simulink model "Thesis_VehicleModel_MPC_ECMS"  (R2018b)
settings: Solver=FixedStepAuto  StartTime=0.0  StopTime=10  FixedStep=0.01  RelTol=1e-5
PostLoadFcn:
  | , if any(exist('dsrtsu_mdlpostloadfcn', 'file') == [2, 3, 6]), try dsrtsu_mdlpostloadfcn('Execute', bdroot); catch fprintf('Error in PostLoadFcn (dsrtsu_mdlpostloadfcn) for model "%s":\n %s\n', bdroot, lasterr); end, end,
InitFcn:
  | clc;clear all;
model workspace (MAT data in the model file):
  MDL : struct (value not decoded)
values from neighbouring files (symbols this model uses):
  MDL =     [MDL.mat]
libraries: simulink x14, rtican x9, autolibshared x1, mpclib x1
(part 5 of 5)

== system Thesis_VehicleModel_MPC_ECMS/Genset Powertrain Dynamics2/Rpm Controller/dSPACE CANBUS Protocol ==
  rpm cmd : Inport
  "rpm " : Inport  Port=2
  DS2202CAN_SETUP_B1_C1 : rtican/RTICAN CONTROLLER SETUP   Reserved1=[]  Reserved2=[]  Reserved3=[]  Reserved4=[]  AcceptanceMask=[]  ArbitrationField=[]  Parameters=[]  SFcnRTICANSettings=[]  MS_Struct=[]  BoardTypeNo=[]  BoardNo=[]  ChannelNo=[]  DialogFcn=[]  UnitName=[]  Revision=[]  UnitValues=[]  DSProperties=struct('RTI',struct('Version',uint32(12),'BlockType',struct('isSLSource',uint8(0),'isSLSink',uint8(0),'isHWSource',uint8(0),'isHWSink',uint8(0),'isSetup',uint8(1),'isInline',uint8(1),'isNonInline',uint8(0),'isInterrupt',uint8(0),'isChannelwise',uint8(0)),'IOBoardType','RTICAN','UnitType','NON_MESSAGE','Identifier','MASTER','DialogType','ML','BlockSet','RTICAN','SlaveProcessor','CAN'))  RTIBlockInterface=struct('InputPortsWidth',int32(0),'InputPortsActive',0,'OutputPortsWidth',int32(0),'OutputPortsActive',0,'DialogFcn','rtican_master_setup_gui','BlockDisplay',{{['CAN CONTROLLER\n SETUP'],'center'}},'IconTransparency','on','InitLevel',3,'IWork',{{{'',uint32(2)}}},'BlockName',struct('Token',{{'DS','CAN_SETUP_B','_C'}},'BlockParam',{{'BoardTypeNo','BoardNo','ChannelNo'}}),'ParameterTunableNames',{{}})  RTIBlockParameters=struct('BoardTypeNo',{{2202,'OFF',[]}},'BoardNo',{{1,'ON',[1 16]}},'ChannelNo',{{1,'ON',[1 2]}},'AcceptanceMask',{{0,'OFF',[]}},'ArbitrationField',{{0,'OFF',[]}},'Parameters',{{struct('Options',struct('DataFileSelected',1,'DataFileName',{{'dbc\dspace_test.dbc'}},'DataFileDate',{{['09-Dec-2018 18:15:36']}},'InterfaceFcn','rtican_dbc_file_parser','InterfaceFcnFileName','','AcceptanceMaskSelected',0,'NumType','hex','MaskType','STD','AcceptanceMask',0,'ArbitrationField',0,'MsgDataType','SgnSpecification','UseMultipleMessageAccess',0),'configType',1,'general',struct('Termination_common',1,'Termination_C252',1,'BusConfigurationRegister',0,'Transceiver','ISO11898','isFromLib',0),'RxReceiveStdOptions',struct('RxServiceStdEnabled',0,'RxServiceStdMsgIdent',1000,'RxServiceStdIdentNumType',1,'RxServiceStdIdentMask',0,'RxServiceStdMaskNumType',1,'RxServiceStdQueueSize',64),'RxReceiveXtdOptions',struct('RxServiceXtdEnabled',0,'RxServiceXtdMsgIdent',1001,'RxServiceXtdIdentNumType',1,'RxServiceXtdIdentMask',0,'RxServiceXtdMaskNumType',1,'RxServiceXtdQueueSize',64),'Config',struct('Baudrate',500,'SampleMode',1,'UsedParamSet',1,'isBTRvalues',0,'validSettings',1,'Advanced',struct('Baudrate',500,'Frequency',36000000,'Settings',struct('SMPL',0,'BRP',1,'NBT',18,'TSEG1',14,'TSEG2',1,'SJW',1,'SP',88),'BTR0',65,'BTR1',30)),'PartialNetworkingOptions',struct('switchedon',0,'format',1,'idmask',['XXXXX XXXXXXXX XXXXXXXX XXXXXXXX'],'idcode','0','idfilter','0','datamaskused',0,'datalength',1,'datamask','0x0000000000000000','partialnetworkenable',0)),'OFF',[]}},'CCPParameters',{{struct('CRO',struct('Format','STD','NumFormat','hex','Id',1639),'DTO',struct('Format','STD','NumFormat','hex','Id',2017),'StationAdr',struct('NumFormat','hex','Value',57),'StationId',struct('Value',['dSPACE CCP Service']),'Enabled',0),'OFF',[]}},'GroupId',{{struct('Group',{{'RTICAN'}},'No',1,'Behavior',{{'EVER'}},'BlockType',{{'SOURCE'}},'NameChangeFlag',1),'OFF',[]}},'SFcnRTICANSettings',{{struct('Baudrate',500,'configType',1,'AdvancedConfig',struct('Frequency',{},'BTR0',{},'BTR1',{}),'UsedParamSet',1,'STDMaskSelected','no','XTDMaskSelected','no','BoardType','DS2202','BoardNo',1,'ControllerNo',1,'Transceiver','ISO11898','BusConfigRegister',0,'TerminationRes',120,'UseMultipleMessageAccess','no','STDRXSrvcUsed','no','STDRXSrvcMsgId',1000,'STDRXSrvcMsgMask',0,'STDRXSrvcQueueSize',64,'XTDRXSrvcUsed','no','XTDRXSrvcMsgId',1001,'XTDRXSrvcQueueSize',64,'XTDRXSrvcMsgMask',0,'PN_IsPNTransciever',0,'PN_IsPNEnabled',0,'PN_MsgFormat',1,'PN_idcode',0,'PN_idmask',2047,'PN_datamaskused',0,'PN_datalength',0,'PN_datamask',['0xFF, 0xFF, 0xFF, 0xFF, 0xFF, 0xFF, 0xFF, 0xFF']),'OFF',[]}},'SFcnRTICCPSettings',{{struct('CRO',struct('Format','STD','NumFormat','hex','Id',1639),'DTO',struct('Format','STD','NumFormat','hex','Id',2017),'StationAdr',struct('NumFormat','hex','Value',57),'StationId',struct('Value',['dSPACE CCP Service']),'Enabled',0),'OFF',[]}},'TLCFileName',{{'rtican_master_setup','OFF',[]}},'XCPParameters',{{struct('MASTER',struct('Format','STD','NumFormat','hex','Id',256),'SLAVE',struct('Format','STD','NumFormat','hex','Id',510),'Enabled',0,'PIDTransmissionEnabled',0),'OFF',[]}},'SFcnRTIXCPSettings',{{struct('MASTER',struct('Format','STD','NumFormat','hex','Id',256),'SLAVE',struct('Format','STD','NumFormat','hex','Id',510),'Enabled',0,'PIDTransmissionEnabled',0),'OFF',[]}})  RTISFcnParameters=struct('SFcnRTICANSettings','struct','SFcnRTICCPSettings','struct','AcceptanceMask','int32','ArbitrationField','int32','TLCFileName','char','SFcnRTIXCPSettings','struct')  RTIBlockParaDefault=struct('BoardTypeNo',4302,'BoardNo',1,'ChannelNo',1,'AcceptanceMask',0,'ArbitrationField',0,'Parameters',struct('Config',{{struct('Baudrate','500','SampleMode',1,'Settings',struct('Frequency',16000000,'BTR0',64,'BTR1',28,'Baudrate',500,'ConfigStruct',struct('Baudrate',500,'Frequency',16000000,'SMPL',0,'BRP',0,'NBT',16,'TSEG1',12,'TSEG2',1,'SJW',1,'SP',87,'BTR0',64,'BTR1',28),'validSettings',1)),struct('Baudrate','500','isBTRvalues',0,'SampleMode',1,'BTR0',64,'BTR1',28,'Settings',struct('Frequency',16000000,'BTR0',128,'BTR1',103,'ListBoxItem',20,'Baudrate',500,'ConfigStruct',struct('Baudrate',500,'Frequency',16000000,'SMPL',0,'BRP',0,'NBT',16,'TSEG1',[12 12 11 11 11 10 10 10 10 9 9 9 9 8 8 8 8 7 7 7 7 6 6 6 6],'TSEG2',[1 1 2 2 2 3 3 3 3 4 4 4 4 5 5 5 5 6 6 6 6 7 7 7 7],'SJW',[0 1 0 1 2 0 1 2 3 0 1 2 3 0 1 2 3 0 1 2 3 0 1 2 3],'SP',[87 87 81 81 81 75 75 75 75 68 68 68 68 62 62 62 62 56 56 56 56 50 50 50 50],'BTR0',[0 64 0 64 128 0 64 128 192 0 64 128 192 0 64 128 192 0 64 128 192 0 64 128 192],'BTR1',[28 28 43 43 43 58 58 58 58 73 73 73 73 88 88 88 88 103 103 103 103 118 118 118 118],'StandardIndex',2),'validSettings',1))}},'Options',struct('DataFileSelected',0,'DataFileName','can_messages.dbc','DataFileDate','','InterfaceFcn','rtican_read_dbc_file','InterfaceFcnFileName','','AcceptanceMaskSelected',0,'NumType','hex','MaskType','STD','AcceptanceMask',0,'ArbitrationField',0),'configType',1,'general',struct('Termination_common',1,'Termination_C252',1,'BusConfigurationRegister',0,'Transceiver','ISO11898','isFromLib',1)),'CCPParameters',struct('CRO',struct('Format','STD','NumFormat','hex','Id',1639),'DTO',struct('Format','STD','NumFormat','hex','Id',2017),'StationAdr',struct('NumFormat','hex','Value',57),'StationId',struct('Value',['dSPACE CCP Service']),'Enabled',0),'GroupId',struct('Group',{{'RTICAN'}},'No',1,'Behavior',{{'EVER'}},'BlockType',{{'SOURCE'}},'NameChangeFlag',1),'SFcnRTICANSettings',struct('Baudrate',500,'Frequency',16000000,'BitTiming0','0x40','BitTiming1','0x1C','STDMaskSelected','no','XTDMaskSelected','no','BoardType','DS4302','BoardNo',1,'ControllerNo',1,'Transceiver','ISO11898','BusConfigRegister',0,'TerminationRes',120),'SFcnRTICCPSettings',struct('CRO',struct('Format','STD','NumFormat','hex','Id',1639),'DTO',struct('Format','STD','NumFormat','hex','Id',2017),'StationAdr',struct('NumFormat','hex','Value',57),'StationId',struct('Value',['dSPACE CCP Service']),'Enabled',0),'TLCFileName','rtican_master_setup','XCPParameters',struct('MASTER',struct('Format','STD','NumFormat','hex','Id',256),'SLAVE',struct('Format','STD','NumFormat','hex','Id',510),'Enabled',0,'PIDTransmissionEnabled',0),'SFcnRTIXCPSettings',struct('MASTER',struct('Format','STD','NumFormat','hex','Id',256),'SLAVE',struct('Format','STD','NumFormat','hex','Id',510),'Enabled',0,'PIDTransmissionEnabled',0))
      settings: AttributesFormatString=Group Id: RTICAN1\n  SourceProductName=dSPACE RTI CAN Blockset
  Data Type Conversion : DataTypeConversion  OutDataTypeStr=int16
  Data Type Conversion1 : DataTypeConversion  OutDataTypeStr=int16
  Data Type Conversion2 : DataTypeConversion  OutDataTypeStr=double
  Terminator{,1..3} (4 alike) : Terminator
  message : rtican/RTICAN Transmit (TX)   Reserved1=[]  Reserved2=[]  Reserved3=[]  Reserved4=[]  SfcnMessage=[]  Msg_Struct=[]  BoardTypeNo=[]  BoardNo=[]  ChannelNo=[]  Parameters=[]  DialogFcn=[]  UnitName=[]  Revision=[]  UnitValues=[]  DSProperties=struct('RTI',struct('Version',uint32(5),'BlockType',struct('isSLSource',uint8(1),'isSLSink',uint8(1),'isHWSource',uint8(0),'isHWSink',uint8(0),'isSetup',uint8(0),'isInline',uint8(1),'isNonInline',uint8(0),'isInterrupt',uint8(0),'isChannelwise',uint8(0)),'IOBoardType','RTICAN','UnitType','MESSAGE','Identifier','TX','DialogType','MSVC','BlockSet','RTICAN','SlaveProcessor','CAN'))  RTIBlockInterface=struct('InputPortsWidth',int32([1 1]),'InputPortsActive',[1 1],'InputPortsName',{{'Eng_rpm','Eng_rpm_Cmd'}},'OutputPortsWidth',int32([1 1]),'OutputPortsActive',[1 1],'OutputPortsName',{{['TX status'],['TX delta time']}},'DialogFcn','rtican_message_interface_gui','BlockDisplay',{{'','center'}},'IconTransparency','on','InitLevel',3,'BlockName',struct('Token',{{'message'}}),'SampleTime',{{0.01}},'TriggerPort',{{'none'}},'EnablePort',{{'none'}},'InputPortsDataType',{{'SS_INT16','SS_INT16'}})  RTIBlockParameters=struct('BoardTypeNo',{{2202,'OFF',[]}},'BoardNo',{{1,'ON',[1 16]}},'ChannelNo',{{1,'ON',[1 2]}},'Parameters',{{struct('DataFileSupport',struct('DataFileSelectedMaster',1,'DataFileSelectedLocal',1,'DataFileName','c:\users\uwecocar3\desktop\yd_thesis_dspace_model\dbc\dspace_test.dbc|','DataFileDate',['10-Dec-2018 12:52:38'],'SelectedFile','dbc\dspace_test.dbc','InterfaceFcn','rtican_dbc_file_parser'),'Options',struct('StatusSelected',1,'TimeSelected',0,'DeltaTimeSelected',1,'DelayTimeSelected',0,'TriggerPort',struct('Selected',0,'TriggerType',0),'EnablePortSelected',0,'SignalOnPortnameSelected',1,'UserCoding',struct('Selected',0,'InterfaceFile','UserEncodingFile','FcnName','UserEncodeFcn','InportSelected',0,'InportWidth',1,'OutportSelected',0,'OutportWidth',1),'TerminationMsg',struct('Selected',0,'Byte0_7','0'),'InitialMsg',struct('Selected',0,'Byte0_7','0'),'DelayTimeTXCommandSelected',0,'EncodeSetUnusedBitsToOne',0,'EnableMsgLoopback',0),'Message',struct('MsgOnBlocknameSelected',1,'MsgName','message','MsgIdFormat',0,'MsgId',16,'MsgLength',4,'NumSignals',2,'SampleTime',0.01,'StartTime',struct('Selected',0,'Value',9),'AutoRepeatTime',struct('Selected',0,'Value',0.1),'Timeout',struct('Selected',0,'Value',0.1),'DelayTime',struct('Selected',0,'Value',0.1),'Signal',struct('SgnName',{'Eng_rpm','Eng_rpm_Cmd'},'SgnStartBit',{0,16},'SgnLength',{16,16},'ByteLayout',{0,0},'Factor',{1,1},'Offset',{0,0},'SgnComment',{'',''},'SgnUnit',{'',''},'Min',{-32768,-32768},'Max',{32767,32767},'SgnType',{0,0},'SLDataType',{'SS_INT16','SS_INT16'},'DataType',{1,1},'ModeValue',{-1,-1}),'MsgIdNumFormat',0,'MsgComment',{{''}}),'Version',1.2,'general',struct('isFromLib',0)),'OFF',[]}},'GroupId',{{struct('Group',{{'RTICAN'}},'No',1,'Behavior',{{'NAMECHANGE'}},'BlockType',{{'SINK'}},'NameChangeFlag',0),'OFF',[]}},'SFcnRTICANMessage',{{struct('MsgType','TX','SFcnPortType','Scalar','MsgName','message','MsgIdFormat','STD','MsgId',16,'MsgLength',4,'NumSignals',2,'SampleTime',0.01,'StartTime',struct('Selected','no','Value',9),'AutoRepeatTime',struct('Selected','no','Value',0.1),'Timeout',struct('Selected','no','Value',0.1),'Signal',struct('SgnName',{'Eng_rpm','Eng_rpm_Cmd'},'SgnStartBit',{0,16},'SgnLength',{16,16},'ByteLayout',{['little endian'],['little endian']},'Factor',{1,1},'Offset',{0,0},'SgnType',{'standard','standard'},'SLDataType',{'SS_INT16','SS_INT16'},'DataType',{['signed int'],['signed int']},'ModeValue',{-1,-1}),'StatusSelected','yes','TimeSelected','no','DeltaTimeSelected','yes','DelayTimeSelected','no','TriggerPort',struct('Selected','no','TriggerType',0),'EnablePortSelected','no','UserCoding',struct('Selected','no','InterfaceFile','UserEncodingFile','FcnName','UserEncodeFcn','InportSelected','no','InportWidth',1,'OutportSelected','no','OutportWidth',1),'TerminationMsg',struct('Selected','no','Byte0','0x00','Byte1','0x00','Byte2','0x00','Byte3','0x00','Byte4','0x00','Byte5','0x00','Byte6','0x00','Byte7','0x00'),'InitialMsg',struct('Selected','no','Byte0','0x00','Byte1','0x00','Byte2','0x00','Byte3','0x00','Byte4','0x00','Byte5','0x00','Byte6','0x00','Byte7','0x00'),'DelayTimeTXCommandSelected','no','EncodeSetUnusedBitsToOne','no','EnableMsgLoopback','no','BoardType','DS2202','BoardNo',1,'ControllerNo',1),'OFF',[]}},'TLCFileName',{{'rtican_tx_message','OFF',[]}})  RTISFcnParameters=struct('SFcnRTICANMessage','struct','TLCFileName','char')  RTIBlockParaDefault=struct('BoardTypeNo',4302,'BoardNo',1,'ChannelNo',1,'Parameters',struct('DataFileSupport',struct('DataFileSelectedMaster',0,'DataFileSelectedLocal',0,'DataFileName','can_messages.dbc','DataFileDate',''),'Options',struct('StatusSelected',1,'TimeSelected',1,'DeltaTimeSelected',1,'DelayTimeSelected',1,'TriggerPort',struct('Selected',0,'TriggerType','rising'),'EnablePortSelected',0,'SignalOnPortnameSelected',1,'UserCoding',struct('Selected',0,'InterfaceFile','UserEncodingFile','FcnName','UserEncodeFcn','InportSelected',0,'InportWidth',1,'OutportSelected',0,'OutportWidth',1),'TerminationMsg',struct('Selected',0,'Byte0_7','0'),'InitialMsg',struct('Selected',0,'Byte0_7','0')),'Message',struct('MsgOnBlocknameSelected',0,'MsgName',['TX Message'],'MsgIdFormat',0,'MsgId',100,'MsgLength',8,'NumSignals',1,'SampleTime',-1,'StartTime',struct('Selected',0,'Value',0),'AutoRepeatTime',struct('Selected',0,'Value',0.1),'Timeout',struct('Selected',0,'Value',0.1),'DelayTime',struct('Selected',0,'Value',0.1),'Signal',struct('SgnName',['TX signal'],'SgnStartBit',0,'SgnLength',8,'SgnType',0,'ModeValue',-1,'DataType',0,'ByteLayout',0,'Factor',1,'Offset',0,'SgnComment',{{}},'SgnUnit',''),'MsgIdNumFormat',0,'MsgComment',{{''}}),'Version',1.2,'general',struct('isFromLib',1)),'GroupId',struct('Group',{{'RTICAN'}},'No',1,'Behavior',{{'NAMECHANGE'}},'BlockType',{{'SINK'}},'NameChangeFlag',0),'SFcnRTICANMessage',struct('MsgType','TX','MsgName',['TX Message'],'MsgIdFormat','STD','MsgId',100,'MsgLength',2,'NumSignals',1,'SampleTime',-1,'StartTime',struct('Selected','no','Value',0),'AutoRepeatTime',struct('Selected','no','Value',0.1),'Timeout',struct('Selected','no','Value',0.1),'DelayTime',struct('Selected','no','Value',0.1),'Signal',struct('SgnName',['TX signal'],'SgnStartBit',0,'SgnLength',8,'SgnType','standard','ModeValue',-1,'DataType',['unsigned int'],'ByteLayout',['little endian'],'Factor',1,'Offset',0),'StatusSelected','yes','TimeSelected','yes','DeltaTimeSelected','yes','DelayTimeSelected','yes','UserCoding',struct('Selected','no','InterfaceFile','UserDecodingFile','FcnName','UserDecodeFcn','InportSelected','no','InportWidth',1,'OutportSelected','no','OutportWidth',1),'TerminationMsg',struct('Selected','no','Byte0','0x00','Byte1','0x00','Byte2','0x00','Byte3','0x00','Byte4','0x00','Byte5','0x00','Byte6','0x00','Byte7','0x00'),'InitialMsg',struct('Selected','no','Byte0','0x00','Byte1','0x00','Byte2','0x00','Byte3','0x00','Byte4','0x00','Byte5','0x00','Byte6','0x00','Byte7','0x00'),'BoardType','DS4302','BoardNo',1,'ControllerNo',1,'SFcnPortType','Scalar'),'TLCFileName','rtican_tx_message')
      settings: AttributesFormatString=Group Id: RTICAN1\n  SourceProductName=dSPACE RTI CAN Blockset
  message_back : rtican/RTICAN Receive (RX)   Reserved1=[]  Reserved2=[]  Reserved3=[]  Reserved4=[]  SfcnMessage=[]  Msg_Struct=[]  BoardTypeNo=[]  BoardNo=[]  ChannelNo=[]  Parameters=[]  DialogFcn=[]  UnitName=[]  Revision=[]  UnitValues=[]  DSProperties=struct('RTI',struct('Version',uint32(5),'BlockType',struct('isSLSource',uint8(1),'isSLSink',uint8(1),'isHWSource',uint8(0),'isHWSink',uint8(0),'isSetup',uint8(0),'isInline',uint8(1),'isNonInline',uint8(0),'isInterrupt',uint8(0),'isChannelwise',uint8(0)),'IOBoardType','RTICAN','UnitType','MESSAGE','Identifier','RX','DialogType','MSVC','BlockSet','RTICAN','SlaveProcessor','CAN'))  RTIBlockInterface=struct('OutputPortsWidth',int32([1 1 1]),'OutputPortsActive',[1 1 1],'OutputPortsName',{{'ThrottleCmd',['RX status'],['RX delta time']}},'OutputPortsLabel',{{'ThrottleCmd','',''}},'OutputPortsLabelMode','ON','InputPortsWidth',int32(1),'InputPortsActive',0,'InputPortsName',{{['User inport']}},'DialogFcn','rtican_message_interface_gui','BlockDisplay',{{'','center'}},'IconTransparency','on','ParameterTunableNames',{{}},'InitLevel',3,'BlockName',struct('Token',{{'message_back'}}),'SampleTime',{{0.01}},'TriggerPort',{{'none'}},'OutputPortsDataType',{{'SS_DOUBLE','SS_DOUBLE','SS_DOUBLE'}},'EnablePort',{{'none'}})  RTIBlockParameters=struct('BoardTypeNo',{{2202,'OFF',[]}},'BoardNo',{{1,'ON',[1 16]}},'ChannelNo',{{1,'ON',[1 2]}},'Parameters',{{struct('DataFileSupport',struct('DataFileSelectedMaster',1,'DataFileSelectedLocal',1,'DataFileName','c:\users\uwecocar3\desktop\yd_thesis_dspace_model\dbc\dspace_test.dbc|','DataFileDate',{{{['10-Dec-2018 12:52:38']}}},'SelectedFile','dbc\dspace_test.dbc','InterfaceFcn','rtican_dbc_file_parser'),'Options',struct('StatusSelected',1,'TimeSelected',0,'DeltaTimeSelected',1,'BytePortSelected',0,'MessageLengthSelected',0,'TriggerPort',struct('Selected',0,'TriggerType',0),'UserCoding',struct('Selected',0,'InterfaceFile','UserDecodingFile','FcnName','UserDecodeFcn','InportSelected',0,'InportWidth',1,'OutportSelected',0,'OutportWidth',1),'EnablePortSelected',0,'SignalOnPortnameSelected',1,'UseRXService',0),'Message',struct('MsgOnBlocknameSelected',1,'MsgName','message_back','MsgIdFormat',0,'MsgId',17,'MsgLength',4,'NumSignals',1,'SampleTime',0.01,'Signal',struct('SgnName','ThrottleCmd','SgnStartBit',0,'SgnLength',16,'SgnType',0,'ModeValue',-1,'DataType',1,'ByteLayout',0,'Factor',3.052e-5,'Offset',0,'SgnComment',{{''}},'SgnUnit','','Min',-1.00007936,'Max',1.00004884,'SLDataType','SS_DOUBLE'),'MsgIdNumFormat',0,'MsgComment',{{''}}),'Version',1.2,'general',struct('isFromLib',0)),'OFF',[]}},'GroupId',{{struct('Group',{{'RTICAN'}},'No',1,'Behavior',{{'NAMECHANGE'}},'BlockType',{{'SINK'}},'NameChangeFlag',0),'OFF',[]}},'SFcnRTICANMessage',{{struct('MsgType','RX','SFcnPortType','Scalar','MsgName','message_back','MsgIdFormat','STD','MsgId',17,'MsgLength',4,'NumSignals',1,'SampleTime',0.01,'Signal',struct('SgnName','ThrottleCmd','SgnStartBit',0,'SgnLength',16,'SgnType','standard','ModeValue',-1,'DataType',['signed int'],'ByteLayout',['little endian'],'Factor',3.052e-5,'Offset',0,'SLDataType','SS_DOUBLE'),'StatusSelected','yes','TimeSelected','no','DeltaTimeSelected','yes','BytePortSelected','no','MessageLengthSelected','no','TriggerPort',struct('Selected','no','TriggerType',0),'UserCoding',struct('Selected','no','InterfaceFile','UserDecodingFile','FcnName','UserDecodeFcn','InportSelected','no','InportWidth',1,'OutportSelected','no','OutportWidth',1),'EnablePortSelected','no','UseRXService','no','BoardType','DS2202','BoardNo',1,'ControllerNo',1),'OFF',[]}},'TLCFileName',{{'rtican_rx_message','OFF',[]}})  RTISFcnParameters=struct('SFcnRTICANMessage','struct','TLCFileName','char')  RTIBlockParaDefault=struct('BoardTypeNo',4302,'BoardNo',1,'ChannelNo',1,'Parameters',struct('DataFileSupport',struct('DataFileSelectedMaster',0,'DataFileSelectedLocal',0,'DataFileName','can_messages.dbc','DataFileDate',''),'Options',struct('StatusSelected',1,'TimeSelected',1,'DeltaTimeSelected',1,'BytePortSelected',0,'MessageLengthSelected',0,'TriggerPort',struct('Selected',0,'TriggerType','rising'),'UserCoding',struct('Selected',0,'InterfaceFile','UserDecodingFile','FcnName','UserDecodeFcn','InportSelected',0,'InportWidth',1,'OutportSelected',0,'OutportWidth',1),'EnablePortSelected',0,'SignalOnPortnameSelected',1),'Message',struct('MsgOnBlocknameSelected',0,'MsgName',['RX Message'],'MsgIdFormat',0,'MsgId',100,'MsgLength',8,'NumSignals',1,'SampleTime',-1,'Signal',struct('SgnName',['RX signal'],'SgnStartBit',0,'SgnLength',8,'SgnType',0,'ModeValue',-1,'DataType',0,'ByteLayout',0,'Factor',1,'Offset',0,'SgnComment',{{}},'SgnUnit',''),'MsgIdNumFormat',0,'MsgComment',{{''}}),'Version',1.2,'general',struct('isFromLib',1)),'GroupId',struct('Group',{{'RTICAN'}},'No',1,'Behavior',{{'NAMECHANGE'}},'BlockType',{{'SINK'}},'NameChangeFlag',0),'SFcnRTICANMessage',struct('MsgType','RX','MsgName',['RX Message'],'MsgIdFormat','STD','MsgId',100,'MsgLength',8,'NumSignals',1,'SampleTime',-1,'Signal',struct('SgnName',['RX signal'],'SgnStartBit',0,'SgnLength',8,'SgnType','standard','ModeValue',-1,'DataType',['unsigned int'],'ByteLayout',['little endian'],'Factor',1,'Offset',0),'StatusSelected','yes','TimeSelected','yes','DeltaTimeSelected','yes','BytePortSelected','no','MessageLengthSelected','no','UserCoding',struct('Selected','no','InterfaceFile','UserDecodingFile','FcnName','UserDecodeFcn','InportSelected','no','InportWidth',1,'OutportSelected','no','OutportWidth',1),'BoardType','DS4302','BoardNo',1,'ControllerNo',1,'SFcnPortType','Scalar'),'TLCFileName','rtican_rx_message')
      settings: AttributesFormatString=Group Id: RTICAN1\n  SourceProductName=dSPACE RTI CAN Blockset
  ThrottleCmd : Outport
  wires:
  message_back/2 -> Terminator/1
  message_back/3 -> Terminator1/1
  message/1 -> Terminator2/1  "TX Status"
  message/2 -> Terminator3/1
  message_back/1 -> Data Type Conversion2/1  "ThrottleCmd"
  rpm cmd/1 -> Data Type Conversion1/1
  "rpm "/1 -> Data Type Conversion/1
  Data Type Conversion/1 -> message/1
  Data Type Conversion1/1 -> message/2
  Data Type Conversion2/1 -> ThrottleCmd/1

== system Thesis_VehicleModel_MPC_ECMS/RTI Data/RTI Data Store/RTI Data Store ==
  RTI Data Store : Subsystem  mask(RTI_DATA_STORE){}
      mask help:
      | RTI Data Store Block. This block is used by RTI to store internal model dependent data. Deleting this block will result in data loss.
      |
      | NEVER DELETE, COPY, OR MODIFY THIS BLOCK!
      mask Help:
      | RTI Data Store Block. This block is used by RTI to store internal model dependent data. Deleting this block will result in data loss.
      | 
      | NEVER DELETE, COPY, OR MODIFY THIS BLOCK!
      mask Display: text(0.5, 0.5, ' ', 'HorizontalAlignment', 'center');

== system Thesis_VehicleModel_MPC_ECMS/Driver and Vehicle Dynamics /Dynamic Model/Three Degree Bicycle Model/Prevent Singularity ==
  In1 : Inport
  Abs : Abs
  Constant : Constant  Value=0.001
  Product : Product
  Sign : Signum
  Switch : Switch  Threshold=0.001
  Switch1 : Switch  Criteria=u2 ~= 0
  Out1 : Outport
  wires:
  In1/1 -> Sign/1, Switch1/2, Switch/1, Abs/1
  Abs/1 -> Switch/2
  Switch/1 -> Switch1/1
  Sign/1 -> Product/1
  Product/1 -> Switch/3
  Switch1/1 -> Out1/1
  Constant/1 -> Switch1/3, Product/2

== system Thesis_VehicleModel_MPC_ECMS/Driver and Vehicle Dynamics /Dynamic Model/Three Degree Bicycle Model/Prevent Singularity1 ==
  In1 : Inport
  Abs : Abs
  Constant : Constant  Value=0.001
  Product : Product
  Sign : Signum
  Switch : Switch  Threshold=0.001
  Switch1 : Switch  Criteria=u2 ~= 0
  Out1 : Outport
  wires:
  In1/1 -> Sign/1, Switch1/2, Switch/1, Abs/1
  Abs/1 -> Switch/2
  Switch/1 -> Switch1/1
  Sign/1 -> Product/1
  Product/1 -> Switch/3
  Switch1/1 -> Out1/1
  Constant/1 -> Switch1/3, Product/2

== system Thesis_VehicleModel_MPC_ECMS/RTI Data/RTI Data Store/RTI Data Store/RTI Data Store ==
  RTI Data Store : Subsystem  mask(RTI_DATA_STORE){}
      mask help:
      | RTI Data Store Block. This block is used by RTI to store internal model dependent data. Deleting this block will result in data loss.
      |
      | NEVER DELETE, COPY, OR MODIFY THIS BLOCK!
      mask Help:
      | RTI Data Store Block. This block is used by RTI to store internal model dependent data. Deleting this block will result in data loss.
      | 
      | NEVER DELETE, COPY, OR MODIFY THIS BLOCK!
      mask Display: text(0.5, 0.5, ' ', 'HorizontalAlignment', 'center');

== system Thesis_VehicleModel_MPC_ECMS/RTI Data/RTI Data Store/RTI Data Store/RTI Data Store/RTI Data Store ==

== matlab function Thesis_VehicleModel_MPC_ECMS/Driver and Vehicle Dynamics /Dynamic Model/Driveline/Fz1 ==
  data: M input; g input; grade input; a input; RearLength input; Length input; CG input; ContactPatch input; EffectiveRadius input; TireInertia input; Faero input; Fz1 output; CD input
function Fz1 = fcn(M,g,grade,a,RearLength,Length,CG,ContactPatch,EffectiveRadius,TireInertia,Faero,CD)

Fzs1 = M*g*RearLength/2/Length;

Fz1 = Fzs1 - 1/2/Length*(M*a*CG + 4*TireInertia*a/EffectiveRadius + Faero * CD +M*g*CG*grade +M*g*ContactPatch);

== matlab function Thesis_VehicleModel_MPC_ECMS/Driver and Vehicle Dynamics /Dynamic Model/Driveline/Fx1 ==
  data: Fz1 input; ContactPatch input; TireInertia input; Fx1 output; EffectiveRadius input; a input
function Fx1 = fcn(Fz1,ContactPatch,TireInertia,EffectiveRadius,a)


Fx1= -(Fz1*ContactPatch + TireInertia*a/EffectiveRadius)/EffectiveRadius;

== matlab function Thesis_VehicleModel_MPC_ECMS/Driver and Vehicle Dynamics /Dynamic Model/Driveline/Fz2 ==
  data: M input; g input; grade input; a input; FrontLength input; Length input; CG input; ContactPatch input; EffectiveRadius input; TireInertia input; Faero input; Fz2 output; CD input
function Fz2 = fcn(M,g,grade,a,FrontLength,Length,CG,ContactPatch,EffectiveRadius,TireInertia,Faero,CD)

Fzs1 = M*g*FrontLength/2/Length;

Fz2 = Fzs1 + 1/2/Length*(M*a*CG + 4*TireInertia*a/EffectiveRadius + Faero * CD +M*g*CG*grade +M*g*ContactPatch);

== stateflow chart Thesis_VehicleModel_MPC_ECMS/Supervisory Control MPC Archive/Chart ==
  state GensetOff
    entry:
    EntryTime = t;
    GensetCmd = MPC_Decision;
  state GensetOn
    entry:
    EntryTime = t;
    GensetCmd = MPC_Decision;
  (default) -> GensetOn
  GensetOn -> GensetOff : [(t - EntryTime > 30) && (GensetCmd != MPC_Decision) ]
  GensetOff -> GensetOn : [(t - EntryTime > 30) && (GensetCmd != MPC_Decision) ]
  data: GensetCmd output double; MPC_Decision input boolean; t input double; EntryTime local double

== matlab function Thesis_VehicleModel_MPC_ECMS/Driver and Vehicle Dynamics /Dynamic Model/Driveline/Explict Transformation ==
  data: M input; g input; grade input; RearLength input; Length input; CG input; ContactPatch input; EffectiveRadius input; Faero input; Fxs output; CD input
function Fxs = fcn(M,g,grade,RearLength,Length,CG,ContactPatch,EffectiveRadius,Faero,CD)

Fzs1 = M*g*RearLength/2/Length;
Coef1 = ContactPatch/2 / EffectiveRadius / Length;

Fxs = -ContactPatch / EffectiveRadius * Fzs1 + Coef1 * (Faero * CD + M*g*CG*grade + M*g *ContactPatch);

== matlab function Thesis_VehicleModel_MPC_ECMS/Driver and Vehicle Dynamics /Dynamic Model/Three Degree Bicycle Model/MATLAB Function1 ==
  data: M input; Denominator output; CG input; WheelInertia input; EffectiveRadius input; Length input; ContactPatch input
function Denominator = fcn(M,CG,WheelInertia,EffectiveRadius,Length,ContactPatch)

Denominator = 1-(1/M* ((ContactPatch/2/EffectiveRadius/Length)*(M * CG  + 4*WheelInertia/EffectiveRadius)...
            - WheelInertia/EffectiveRadius^2));
end

== matlab function Thesis_VehicleModel_MPC_ECMS/Driver and Vehicle Dynamics /Dynamic Model/Driveline/Front Lateral Force Characteristic Function (Linear Model without Relexation) ==
  data: SlipAngle input; Y_alpha1 output; Caf input
function Y_alpha1 = fcn(SlipAngle,Caf)

Y_alpha1 = Caf*SlipAngle;
end

== matlab function Thesis_VehicleModel_MPC_ECMS/Driver and Vehicle Dynamics /Dynamic Model/Driveline/Rear Lateral Force Characteristic Function (Linear Model without Relexation) ==
  data: SlipAngle input; Y_alpha2 output; Car input
function Y_alpha2 = fcn(SlipAngle,Car)

Y_alpha2 =Car * SlipAngle;
end

== matlab function Thesis_VehicleModel_MPC_ECMS/Driver and Vehicle Dynamics /Dynamic Model/Three Degree Bicycle Model/Compute Global Velocity ==
  data: Yaw input; v input; u input; Xdot output; Ydot output
function [Xdot,Ydot] = fcn(Yaw,v,u)

Xdot = u*cos(Yaw) -v*sin(Yaw);
Ydot = u*sin(Yaw) +v*cos(Yaw);

== matlab function Thesis_VehicleModel_MPC_ECMS/Driver and Vehicle Dynamics /Dynamic Model/Three Degree Bicycle Model/MATLAB Function ==
  data: Xdot input; V output; Ydot input
function V = fcn(Xdot,Ydot)

V = norm([Xdot,Ydot]);

== matlab function Thesis_VehicleModel_MPC_ECMS/Driver and Vehicle Dynamics /Dynamic Model/Three Degree Bicycle Model/Aero Resistance ==
  data: u input; Faero output; Rho input; CdA input
function Faero = fcn(u,Rho,CdA)


Faero = 0.5 * Rho * CdA * u^2;

== stateflow chart Thesis_VehicleModel_MPC_ECMS/Genset Powertrain Dynamics/Rpm Controller/rpm regulation ==
  state Initialize
    entry:
    EntryTime = t;
    rpm_ref_update = rpm_ref;
  state rpmUpdate
    entry:
    EntryTime = t;
    rpm_ref_update = rpm;
  state rpmUpdate1
    entry:
    EntryTime = t;
    rpm_ref_update = rpm;
  (default) -> Initialize
  rpmUpdate -> Initialize [order 2] : [hasChanged(rpm_ref)||hasChanged(GensetOnOff)]
  rpmUpdate1 -> Initialize [order 2] : [hasChanged(rpm_ref)||hasChanged(GensetOnOff)]
  Initialize -> rpmUpdate : [((t - EntryTime) > 10) && (abs(rpm_ref_update - rpm)>=100)]
  rpmUpdate -> rpmUpdate1 [order 1] : [((t - EntryTime) > 10) && (abs(rpm_ref_update - rpm)>=100)]
  rpmUpdate1 -> rpmUpdate [order 1] : [((t - EntryTime) > 10) && (abs(rpm_ref_update - rpm)>=100)]
  data: rpm input; rpm_ref input; EntryTime local double; t input double; rpm_ref_update output double; GensetOnOff input double

== matlab function Thesis_VehicleModel_MPC_ECMS/Genset Powertrain Dynamics/Power//rpm Setpoints/MATLAB Function ==
  data: Power_Cmd input; PowerSetPoint output; rpmSetPoint output; GensetCmd input
function [PowerSetPoint,rpmSetPoint] = fcn(Power_Cmd,GensetCmd)

if GensetCmd == 0
    PowerSetPoint = 0;
    rpmSetPoint = 0;
else
    if Power_Cmd >=25000
        PowerSetPoint = 25000;
        rpmSetPoint = 4000;
    elseif Power_Cmd >= 20000
        PowerSetPoint = 20000;
        rpmSetPoint = 3500;
    else
        PowerSetPoint = 10000;
        rpmSetPoint = 2500;
    end
end

== matlab function Thesis_VehicleModel_MPC_ECMS/Genset Powertrain Dynamics/Rpm Controller/LQG Gain Mapping ==
  data: comp output; gain output; rpm input; rpm_cmd input; PowerSetPoint input
function [comp,gain] = fcn(rpm,rpm_cmd,PowerSetPoint)
gain = -[ 0.1124 ,0.1082];

if rpm_cmd == 2500
    comp = - (55+27.5904-13.09)/132;
elseif rpm_cmd == 3500
    comp = -(60+34.1185-18.3260)/140;
elseif rpm_cmd == 4000
    comp = -(63+37.8922-20.9440)/142;
else
    comp = 0;
end

== matlab function Thesis_VehicleModel_MPC_ECMS/Genset Powertrain Dynamics/Rpm Controller/Kalman Filter/Bu ==
  data: u input; y output; Tmax input
function y = fcn(u,Tmax)

B = [0;Tmax/(0.2*0.73)];
y = B*u;

== matlab function Thesis_VehicleModel_MPC_ECMS/Genset Powertrain Dynamics/Generator/Voltage, Current and Load Torque Mapping ==
  data: P input; Volt output; Current output; LoadTorque output
function [Volt,Current,LoadTorque] = fcn(P)
if P == 10000
    Volt = 340;
    Current = P/340;
    LoadTorque = 55;
elseif P == 20000
    Volt = 340;
    Current = P/340;
    LoadTorque = 60; 
elseif P == 25000
    Volt = 420;
    Current = 25000/420;
    LoadTorque = 63; 
else
    Volt = 340;
    Current = 0;
    LoadTorque = 0;
end

== stateflow chart Thesis_VehicleModel_MPC_ECMS/Genset Powertrain Dynamics/Power//rpm Setpoints/Chart ==
  state CmdHold1
    entry:
    EntryTime = t;
    rpmCmd = rpmSetPoint;
    PowerCmd = PowerSetPoint;
  state CmdHold
    entry:
    EntryTime = t;
    rpmCmd = rpmSetPoint;
    PowerCmd = PowerSetPoint;
  (default) -> CmdHold
  CmdHold -> CmdHold1 : [(t - EntryTime > 30) ]
  CmdHold1 -> CmdHold : [(t - EntryTime > 30) ]
  data: PowerSetPoint input double; t input double; EntryTime local double; rpmSetPoint input double; rpmCmd output double; PowerCmd output double

== matlab function Thesis_VehicleModel_MPC_ECMS/Genset Powertrain Dynamics/Engine/Engine_Dynamics /Closed throttle torque ==
  data: w input; T output
function T = Tcct(w)
if w == 0
    T_init = -10;
else
    T_init = 0;
end

omega = w*30/pi;
T = T_init-17.27-28.99*(omega/12000) - 98.63*(omega/12000)^2;
end

== matlab function Thesis_VehicleModel_MPC_ECMS/Driver and Vehicle Dynamics /EMRAX Motor Model /EMRAX 228 Motor/Spin Loss  ==
  data: omega input; T_sl output
function T_sl = Spinloss(omega)

T_damp = 5;
T_sl = sign(omega)*(- 2.8 *(omega/12000) - T_damp);

== matlab function Thesis_VehicleModel_MPC_ECMS/Supervisory Control ECMS/MATLAB Function ==
  data: Preq input; Peng output; SOCt input; Qlhv input; Qbatt input; SOCmax input; SOCmin input; SOCref input; a input; R input; MinCost output
function [Peng,MinCost] = fcn(Preq,SOCt,Qlhv,Qbatt,SOCmax,SOCmin,SOCref,a,R)
%% Parameter Config
d = (SOCmax - SOCmin)/2;
P_eng = 0:1000:25000;
p_SOC = 1 - ((SOCt - SOCref)/d)^a;
Lambda = -2.5e3;
%% Estimate Engine Efficiency via Quadratic function 
C0 = 6760;C1 = 2.17805387584195;C2 = 1.23361230213725e-06;      % Coefficiencts of Power loss of engine
P_eng_loss = C0 + C1.*P_eng + C2*P_eng.^2;
%% Search for Optimal Candidate 
P_batt = Preq - P_eng;                                           % ith candidate: P_eng + P_batt = Preq
%Compute equivalence factor
a2 = 0.00294542788994159;b2 = 1.73706104317792;                           % Linear Interp of Current 
I = a2.*P_batt + b2;
Eta_bar = P_batt ./ (340*I);                                     % Make sure it is the same lambda in CusCost
s = -Qlhv./Eta_bar/Qbatt*Lambda;
%Compute different candidates
Fuel_Comsp = (P_eng+P_eng_loss)/Qlhv;
Eqv_Fuel_Comsp = P_batt.*s/Qlhv * p_SOC;
Candidate = Fuel_Comsp + Eqv_Fuel_Comsp;
    
%% Decide Optimal Candidate
[MinCost,Index] = min(Candidate);
% FC_Optimal = (P_eng(Index) + P_eng_loss(Index))/Qlhv
% Eqv_FC_Optimal = P_batt(Index) * s(Index) / Qlhv * p_SOC
Peng = P_eng(Index);

== matlab function Thesis_VehicleModel_MPC_ECMS/Genset Powertrain Dynamics1/Engine/Engine_Dynamics /Closed throttle torque ==
  data: w input; T output
function T = Tcct(w)
if w == 0
    T_init = -10;
else
    T_init = 0;
end

omega = w*30/pi;
T = T_init-17.27-28.99*(omega/12000) - 98.63*(omega/12000)^2;
end

== matlab function Thesis_VehicleModel_MPC_ECMS/Genset Powertrain Dynamics1/Generator/Voltage, Current and Load Torque Mapping ==
  data: P input; Volt output; Current output; LoadTorque output
function [Volt,Current,LoadTorque] = fcn(P)
if P == 10000
    Volt = 340;
    Current = P/340;
    LoadTorque = 55;
elseif P == 20000
    Volt = 340;
    Current = P/340;
    LoadTorque = 60; 
elseif P == 25000
    Volt = 420;
    Current = 25000/420;
    LoadTorque = 63; 
else
    Volt = 340;
    Current = 0;
    LoadTorque = 0;
end

== stateflow chart Thesis_VehicleModel_MPC_ECMS/Genset Powertrain Dynamics1/Power//rpm Setpoints/Chart ==
  state CmdHold1
    entry:
    EntryTime = t;
    rpmCmd = rpmSetPoint;
    PowerCmd = PowerSetPoint;
  state CmdHold
    entry:
    EntryTime = t;
    rpmCmd = rpmSetPoint;
    PowerCmd = PowerSetPoint;
  (default) -> CmdHold
  CmdHold -> CmdHold1 : [(t - EntryTime > 30) ]
  CmdHold1 -> CmdHold : [(t - EntryTime > 30) ]
  data: PowerSetPoint input double; t input double; EntryTime local double; rpmSetPoint input double; rpmCmd output double; PowerCmd output double

== matlab function Thesis_VehicleModel_MPC_ECMS/Genset Powertrain Dynamics1/Power//rpm Setpoints/MATLAB Function ==
  data: Power_Cmd input; PowerSetPoint output; rpmSetPoint output; GensetCmd input
function [PowerSetPoint,rpmSetPoint] = fcn(Power_Cmd,GensetCmd)

if GensetCmd == 0
    PowerSetPoint = 0;
    rpmSetPoint = 0;
else
    if Power_Cmd >=25000
        PowerSetPoint = 25000;
        rpmSetPoint = 4000;
    elseif Power_Cmd >= 20000
        PowerSetPoint = 20000;
        rpmSetPoint = 3500;
    else
        PowerSetPoint = 10000;
        rpmSetPoint = 2500;
    end
end

== matlab function Thesis_VehicleModel_MPC_ECMS/Genset Powertrain Dynamics1/Rpm Controller/Kalman Filter/Bu ==
  data: u input; y output; Tmax input
function y = fcn(u,Tmax)

B = [0;Tmax/(0.2*0.73)];
y = B*u;

== matlab function Thesis_VehicleModel_MPC_ECMS/Genset Powertrain Dynamics1/Rpm Controller/LQG Gain Mapping ==
  data: comp output; gain output; rpm input; rpm_cmd input; PowerSetPoint input
function [comp,gain] = fcn(rpm,rpm_cmd,PowerSetPoint)
gain = -[ 0.1124 ,0.1082];

if rpm_cmd == 2500
    comp = - (55+27.5904-13.09)/132;
elseif rpm_cmd == 3500
    comp = -(60+34.1185-18.3260)/140;
elseif rpm_cmd == 4000
    comp = -(63+37.8922-20.9440)/142;
else
    comp = 0;
end

== stateflow chart Thesis_VehicleModel_MPC_ECMS/Genset Powertrain Dynamics1/Rpm Controller/rpm regulation ==
  state Initialize
    entry:
    EntryTime = t;
    rpm_ref_update = rpm_ref;
  state rpmUpdate
    entry:
    EntryTime = t;
    rpm_ref_update = rpm;
  state rpmUpdate1
    entry:
    EntryTime = t;
    rpm_ref_update = rpm;
  (default) -> Initialize
  rpmUpdate -> Initialize [order 2] : [hasChanged(rpm_ref)||hasChanged(GensetOnOff)]
  rpmUpdate1 -> Initialize [order 2] : [hasChanged(rpm_ref)||hasChanged(GensetOnOff)]
  Initialize -> rpmUpdate : [((t - EntryTime) > 10) && (abs(rpm_ref_update - rpm)>=100)]
  rpmUpdate -> rpmUpdate1 [order 1] : [((t - EntryTime) > 10) && (abs(rpm_ref_update - rpm)>=100)]
  rpmUpdate1 -> rpmUpdate [order 1] : [((t - EntryTime) > 10) && (abs(rpm_ref_update - rpm)>=100)]
  data: rpm input; rpm_ref input; EntryTime local double; t input double; rpm_ref_update output double; GensetOnOff input double

== stateflow chart Thesis_VehicleModel_MPC_ECMS/Supervisory Control ECMS/Chart ==
  state GensetOff
    entry:
    EntryTime = t;
    GensetCmd = MPC_Decision;
  state GensetOn
    entry:
    EntryTime = t;
    GensetCmd = MPC_Decision;
  (default) -> GensetOn
  GensetOn -> GensetOff : [(t - EntryTime > 30) && (GensetCmd != MPC_Decision) ]
  GensetOff -> GensetOn : [(t - EntryTime > 30) && (GensetCmd != MPC_Decision) ]
  data: GensetCmd output double; MPC_Decision input boolean; t input double; EntryTime local double

== matlab function Thesis_VehicleModel_MPC_ECMS/Solve One-Step QP Problem/A1 ==
  data: SOC input; A1 output; SOC_ref input; Qbatt input; SOC_max input; SOC_min input; Voltage input
function A1 = fcn(SOC,SOC_ref,Qbatt,SOC_max,SOC_min,Voltage)
d = (SOC_max - SOC_min)/2;
a = 0.00294542788994159;b = 1.73706104317792; % 1st order Current Approximation  
Delta_SOC = SOC - SOC_ref;
Lambda = - 2e3;
A1 = - Lambda* (1 - Delta_SOC / d) * a*Voltage * (1/Qbatt);

== matlab function Thesis_VehicleModel_MPC_ECMS/Solve One-Step QP Problem/B1, B2 ==
  data: Qlhv input; B1 output; Preq input; B2 output
function [B1,B2] = fcn(Qlhv,Preq)

C0 = 6760;C1 = 2.17805387584195;C2 = 1.23361230213725e-06;  % Power loss approximation
B1 = 1/Qlhv * (-C1 -1 -2 * C2 * Preq);
B2 = C2/Qlhv;

== stateflow chart Thesis_VehicleModel_MPC_ECMS/Solve One-Step QP Problem/Chart ==
  state GensetOff
    entry:
    EntryTime = t;
    GensetCmd = MPC_Decision;
  state GensetOn
    entry:
    EntryTime = t;
    GensetCmd = MPC_Decision;
  (default) -> GensetOn
  GensetOn -> GensetOff : [(t - EntryTime > 30) && (GensetCmd != MPC_Decision) ]
  GensetOff -> GensetOn : [(t - EntryTime > 30) && (GensetCmd != MPC_Decision) ]
  data: GensetCmd output double; MPC_Decision input boolean; t input double; EntryTime local double

== matlab function Thesis_VehicleModel_MPC_ECMS/Solve One-Step QP Problem/MATLAB Function ==
  settings: sampleTime=1
  data: Preq input; SOC_0 input; x1 output size=1; x2 output; x3 output; SOC_ref input; SOC_max input; SOC_min input; Peng_min input; Peng_max input; Qbatt input; iA input boolean; status output; iA1 output
function [x1,x2,x3,status,iA1] = MPC(Preq,SOC_0,SOC_ref,SOC_max,SOC_min,Peng_min,Peng_max,Qbatt,iA)
%% Construct Problem: min J = 1/2 x'Hx + F'x; s.t. Ac'x >= b0, Aeq'x = beq.
lambda = -2.5e3;
d = (SOC_max - SOC_min)/2;
delSOC = SOC_0 - SOC_ref;
w1 = lambda * (1 - delSOC/d);
w2 = 1/44400;
d1 = [1,0,0]; d2 = [0,1,0];d3 = [0,0,1];
a1 = 0.00294542788994159;a0 = 1.73706104317792;               % 1st order Current Approximation  
C1 = 2.17805387584195;C2 = 1.23361230213725e-06;    % Engine Power loss approximation
% Construct Parameter for mpcsolver
H = w2*C2*diag([0.0001,1,0.000001])*2;
L = chol(H, 'lower');
Linv = L\eye(size(H,1));
F = w1*d1 + w2*(C1+1)*d2;                               % J = 1/2 x'Hx + f'x, x = [SOC,Peng,Pbatt]
aeq_1 = d1 + (340*a1/Qbatt)*d3;                     % Equality Const 1: Dynamics
beq_1 = -340/Qbatt*a0 + SOC_0;
aeq_2 = [0,1,1];                                    % Equality Const 2: Power Equality
beq_2 = Preq;
Aeq = [aeq_1;aeq_2];beq = [beq_1;beq_2];            % Equality Constraint
Aineq = [d1;d2;-d1;-d2]; 
bineq = [SOC_min;Peng_min;-SOC_max;-Peng_max];      % Inequality Constraint
%#codegen
opt = mpcqpsolverOptions;
[u, status,iA1] = mpcqpsolver(Linv, F', Aineq, bineq,Aeq, beq, iA ,opt);
x1 = u(1);x2 = u(2);x3 = u(3);

== matlab function Thesis_VehicleModel_MPC_ECMS/Solve Multiple-Step QP Problem/MPC Problem 2 ==
  settings: sampleTime=1
  data: Preq input; SOC_0 input; x1 output size=[5,1]; x2 output size=[5,1]; x3 output size=[5,1]; SOC_ref input; SOC_max input; SOC_min input; Peng_min input; Peng_max input; Qbatt input; status output; iA input boolean; iA1 output
function [x1,x2,x3,status,iA1] = MPC(Preq,SOC_0,SOC_ref,SOC_max,SOC_min,Peng_min,Peng_max,Qbatt,iA)
%% Construct Problem: min J = 1/2 x'Hx + F'x; s.t. Ac'x >= b0, Aeq'x = beq.
T = 5;
lambda = -2.5e3;
d = (SOC_max - SOC_min)/2;
delSOC = SOC_0 - SOC_ref;
w1 = abs(lambda * (1 - delSOC/d));
w2 = 1/44400;                                               % Weights of obj fcn
I = eye(T);
d1 = [I,zeros(T),zeros(T),zeros(T,1)]; 
d2 = [zeros(T),I,zeros(T),zeros(T,1)];
d3 = [zeros(T),zeros(T),I,zeros(T,1)];
c1 = [I,zeros(T),zeros(T),ones(T,1)]; 
c2 = [-I,zeros(T),zeros(T),ones(T,1)];                      % Construct vectors
a1 = 0.00294542788994159;a0 = 1.73706104317792;             % 1st order Current Approximation  
C1 = 2.17805387584195;C2 = 1.23361230213725e-06;            % Engine Power loss approximation
%% Construct Parameter for mpcsolver
Miu = 0.0001;
H = w2*C2*diag([Miu*ones(1,T),ones(1,T),Miu*ones(1,T),Miu])*2;
L = chol(H, 'lower');
Linv = L\eye(size(H,1));
F = w1*[zeros(1,3*T),1] + w2*(C1+1)*ones(1,T)*d2;           % J = 1/2 x'Hx + F'x, x = [SOC,Peng,Pbatt,t]
aeq_1 = d1 + (340*a1/Qbatt)*tril(ones(T,T))*d3;             % Equality Const 1: Dynamics
beq_1 = (-340/Qbatt*a0 + SOC_0)*ones(T,1);
aeq_2 = [zeros(T),eye(T),eye(T),zeros(T,1)];                         % Equality Const 2: Power Equality
beq_2 = linspace(Preq,0,T);
Aeq = [aeq_1;aeq_2];beq = [beq_1;beq_2'];                   % Equality Constraint
Aineq = [d1;d2;-d1;-d2;c1;c2]; 
bineq = [SOC_min*ones(T,1);
        Peng_min*ones(T,1);
        -SOC_max*ones(T,1);
        -Peng_max*ones(T,1);
        SOC_ref*ones(T,1);
        -SOC_ref*ones(T,1)];                                % Inequality Constraint
%#codegen
opt = mpcqpsolverOptions;
[u, status,iA1] = mpcqpsolver(Linv, F', Aineq, bineq,Aeq, beq, iA ,opt);
x1 = u(1:T);x2 = u(T+1:2*T);x3 = u(2*T+1:3*T);

== matlab function Thesis_VehicleModel_MPC_ECMS/Driver and Vehicle Dynamics /EMRAX Motor Model /EMRAX 228 Motor/MATLAB Function ==
  data: Eff input; P_mot input; Efficiency output
function Efficiency = fcn(Eff,P_mot)

if P_mot >=0
    Efficiency = Eff;
else
    Efficiency = 1/Eff;
end

== stateflow chart Thesis_VehicleModel_MPC_ECMS/Solve Multiple-Step QP Problem/Chart ==
  state GensetOff
    entry:
    EntryTime = t;
    GensetCmd = MPC_Decision;
  state GensetOn
    entry:
    EntryTime = t;
    GensetCmd = MPC_Decision;
  (default) -> GensetOn
  GensetOn -> GensetOff : [(t - EntryTime > 30) && (GensetCmd != MPC_Decision) ]
  GensetOff -> GensetOn : [(t - EntryTime > 30) && (GensetCmd != MPC_Decision) ]
  data: GensetCmd output double; MPC_Decision input boolean; t input double; EntryTime local double

== matlab function Thesis_VehicleModel_MPC_ECMS/Solve Multiple-Step QP Problem/MPC Problem 1 ==
  settings: sampleTime=1
  data: Preq input; SOC_0 input; x1 output size=[5,1]; x2 output size=[5,1]; x3 output size=[5,1]; SOC_ref input; SOC_max input; SOC_min input; Peng_min input; Peng_max input; Qbatt input; status output; iA input boolean; iA1 output
function [x1,x2,x3,status,iA1] = MPC(Preq,SOC_0,SOC_ref,SOC_max,SOC_min,Peng_min,Peng_max,Qbatt,iA)
%% Construct Problem: min J = 1/2 x'Hx + F'x; s.t. Ac'x >= b0, Aeq'x = beq.
T = 5;
lambda = -2e2/4;
d = (SOC_max - SOC_min)/2;
delSOC = SOC_0 - SOC_ref;
w1 = lambda * (1 - delSOC/d);
w2 = 1/44400;
I = eye(T);
d1 = [I,zeros(T),zeros(T)]; d2 = [zeros(T),I,zeros(T)];d3 = [zeros(T),zeros(T),I];
a1 = 0.030; a0 = -0.321256961515499;                % 1st order Current Approximation  
C1 = 2.17805387584195;C2 = 1.23361230213725e-06;    % Engine Power loss approximation
% Construct Parameter for mpcsolver
Miu = 0.0001;
H = w2*C2*diag([Miu*ones(1,T),ones(1,T),Miu*ones(1,T)])*2;
L = chol(H, 'lower');
Linv = L\eye(size(H,1));
F = w1*ones(1,T)*d1 + w2*(C1+1)*ones(1,T)*d2;                               % J = 1/2 x'Hx + f'x, x = [SOC,Peng,Pbatt]
aeq_1 = d1 + (340*a1/Qbatt)*tril(ones(T,T))*d3;                     % Equality Const 1: Dynamics
beq_1 = (-340/Qbatt*a0 + SOC_0)*ones(T,1);
aeq_2 = [zeros(T),eye(T),eye(T)];                                    % Equality Const 2: Power Equality
beq_2 = linspace(Preq,0,T);
Aeq = [aeq_1;aeq_2];beq = [beq_1;beq_2'];            % Equality Constraint
Aineq = [d1;d2;-d1;-d2]; 
bineq = [SOC_min*ones(T,1);Peng_min*ones(T,1);-SOC_max*ones(T,1);-Peng_max*ones(T,1)];      % Inequality Constraint
%#codegen
opt = mpcqpsolverOptions;
[u, status,iA1] = mpcqpsolver(Linv, F', Aineq, bineq,Aeq, beq, iA ,opt);
x1 = u(1:T);x2 = u(T+1:2*T);x3 = u(2*T+1:3*T);

== matlab function Thesis_VehicleModel_MPC_ECMS/Genset Powertrain Dynamics2/Engine/Engine_Dynamics /Closed throttle torque ==
  data: w input; T output
function T = Tcct(w)
if w == 0
    T_init = -10;
else
    T_init = 0;
end

omega = w*30/pi;
T = T_init-17.27-28.99*(omega/12000) - 98.63*(omega/12000)^2;
end

== matlab function Thesis_VehicleModel_MPC_ECMS/Genset Powertrain Dynamics2/Generator/Voltage, Current and Load Torque Mapping ==
  data: P input; Volt output; Current output; LoadTorque output
function [Volt,Current,LoadTorque] = fcn(P)
if P == 10000
    Volt = 340;
    Current = P/340;
    LoadTorque = 55;
elseif P == 20000
    Volt = 340;
    Current = P/340;
    LoadTorque = 60; 
elseif P == 25000
    Volt = 420;
    Current = 25000/420;
    LoadTorque = 63; 
else
    Volt = 340;
    Current = 0;
    LoadTorque = 0;
end

== stateflow chart Thesis_VehicleModel_MPC_ECMS/Genset Powertrain Dynamics2/Power//rpm Setpoints/Chart ==
  state CmdHold1
    entry:
    EntryTime = t;
    rpmCmd = rpmSetPoint;
    PowerCmd = PowerSetPoint;
  state CmdHold
    entry:
    EntryTime = t;
    rpmCmd = rpmSetPoint;
    PowerCmd = PowerSetPoint;
  (default) -> CmdHold
  CmdHold -> CmdHold1 : [(t - EntryTime > 30) ]
  CmdHold1 -> CmdHold : [(t - EntryTime > 30) ]
  data: PowerSetPoint input double; t input double; EntryTime local double; rpmSetPoint input double; rpmCmd output double; PowerCmd output double

== matlab function Thesis_VehicleModel_MPC_ECMS/Genset Powertrain Dynamics2/Power//rpm Setpoints/MATLAB Function ==
  data: Power_Cmd input; PowerSetPoint output; rpmSetPoint output; GensetCmd input
function [PowerSetPoint,rpmSetPoint] = fcn(Power_Cmd,GensetCmd)

if GensetCmd == 0
    PowerSetPoint = 0;
    rpmSetPoint = 0;
else
    if Power_Cmd >=25000
        PowerSetPoint = 25000;
        rpmSetPoint = 4000;
    elseif Power_Cmd >= 20000
        PowerSetPoint = 20000;
        rpmSetPoint = 3500;
    else
        PowerSetPoint = 10000;
        rpmSetPoint = 2500;
    end
end

== matlab function Thesis_VehicleModel_MPC_ECMS/Genset Powertrain Dynamics2/Rpm Controller/Kalman Filter/Bu ==
  data: u input; y output; Tmax input
function y = fcn(u,Tmax)

B = [0;Tmax/(0.2*0.73)];
y = B*u;

== matlab function Thesis_VehicleModel_MPC_ECMS/Genset Powertrain Dynamics2/Rpm Controller/LQG Gain Mapping ==
  data: comp output; gain output; rpm input; rpm_cmd input; PowerSetPoint input
function [comp,gain] = fcn(rpm,rpm_cmd,PowerSetPoint)
gain = -[ 0.1124 ,0.1082];

if rpm_cmd == 2500
    comp = - (55+27.5904-13.09)/132;
elseif rpm_cmd == 3500
    comp = -(60+34.1185-18.3260)/140;
elseif rpm_cmd == 4000
    comp = -(63+37.8922-20.9440)/142;
else
    comp = 0;
end

== stateflow chart Thesis_VehicleModel_MPC_ECMS/Genset Powertrain Dynamics2/Rpm Controller/rpm regulation ==
  state Initialize
    entry:
    EntryTime = t;
    rpm_ref_update = rpm_ref;
  state rpmUpdate
    entry:
    EntryTime = t;
    rpm_ref_update = rpm;
  state rpmUpdate1
    entry:
    EntryTime = t;
    rpm_ref_update = rpm;
  (default) -> Initialize
  rpmUpdate -> Initialize [order 2] : [hasChanged(rpm_ref)||hasChanged(GensetOnOff)]
  rpmUpdate1 -> Initialize [order 2] : [hasChanged(rpm_ref)||hasChanged(GensetOnOff)]
  Initialize -> rpmUpdate : [((t - EntryTime) > 10) && (abs(rpm_ref_update - rpm)>=100)]
  rpmUpdate -> rpmUpdate1 [order 1] : [((t - EntryTime) > 10) && (abs(rpm_ref_update - rpm)>=100)]
  rpmUpdate1 -> rpmUpdate [order 1] : [((t - EntryTime) > 10) && (abs(rpm_ref_update - rpm)>=100)]
  data: rpm input; rpm_ref input; EntryTime local double; t input double; rpm_ref_update output double; GensetOnOff input double
